simulink model "TST_CoPT_TrqLeadCoord"  (R2016b)
settings: Solver=FixedStepDiscrete  StartTime=0.0  StopTime=simTime  FixedStep=sampleTime  RelTol=1e-3
values from neighbouring files (symbols this model uses):
  testCase = 1    [initTST_CoPT_TrqLeadCoord_001.m]    (also in initTST_CoPT_TrqLeadCoord_002.m = 2)
libraries: simulink x9, UnitTest_Lib x6
settings Model: Creator=zhengjinyan  LastModifiedBy=zhengjinyan
settings DebuggingCC: SignalRangeChecking=error

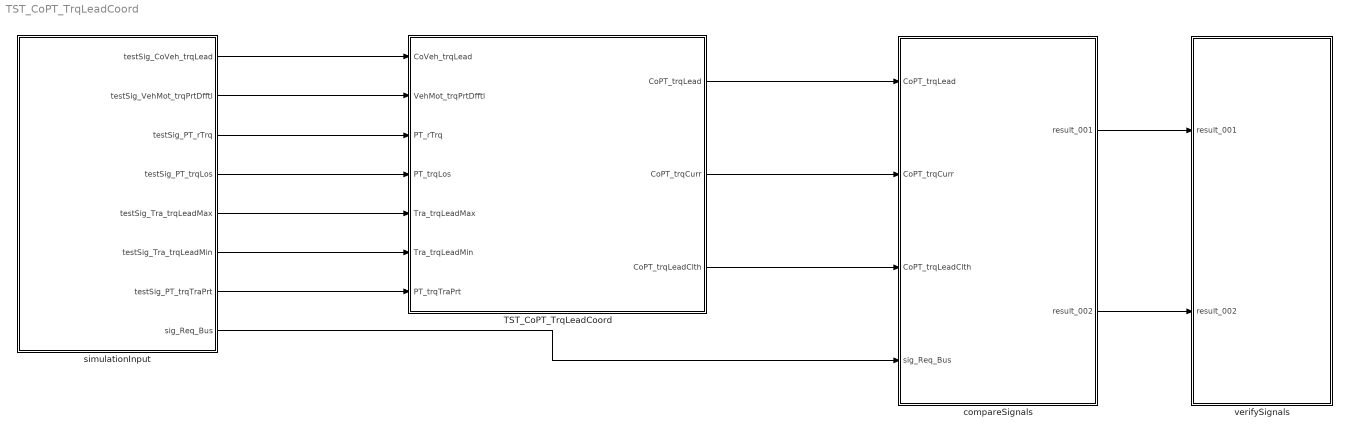
== system TST_CoPT_TrqLeadCoord ==
  TST_CoPT_TrqLeadCoord : Subsystem
  compareSignals : Subsystem
  simulationInput : Subsystem
  verifySignals : Subsystem
  wires:
  simulationInput/1(testSig_CoVeh_trqLead) -> TST_CoPT_TrqLeadCoord/1(CoVeh_trqLead)
  simulationInput/2(testSig_VehMot_trqPrtDfftl) -> TST_CoPT_TrqLeadCoord/2(VehMot_trqPrtDfftl)
  simulationInput/3(testSig_PT_rTrq) -> TST_CoPT_TrqLeadCoord/3(PT_rTrq)
  simulationInput/4(testSig_PT_trqLos) -> TST_CoPT_TrqLeadCoord/4(PT_trqLos)
  simulationInput/5(testSig_Tra_trqLeadMax) -> TST_CoPT_TrqLeadCoord/5(Tra_trqLeadMax)
  simulationInput/6(testSig_Tra_trqLeadMin) -> TST_CoPT_TrqLeadCoord/6(Tra_trqLeadMin)
  simulationInput/7(testSig_PT_trqTraPrt) -> TST_CoPT_TrqLeadCoord/7(PT_trqTraPrt)
  TST_CoPT_TrqLeadCoord/1(CoPT_trqLead) -> compareSignals/1(CoPT_trqLead)
  TST_CoPT_TrqLeadCoord/2(CoPT_trqCurr) -> compareSignals/2(CoPT_trqCurr)
  TST_CoPT_TrqLeadCoord/3(CoPT_trqLeadClth) -> compareSignals/3(CoPT_trqLeadClth)
  simulationInput/8(sig_Req_Bus) -> compareSignals/4(sig_Req_Bus)
  compareSignals/1(result_001) -> verifySignals/1(result_001)
  compareSignals/2(result_002) -> verifySignals/2(result_002)

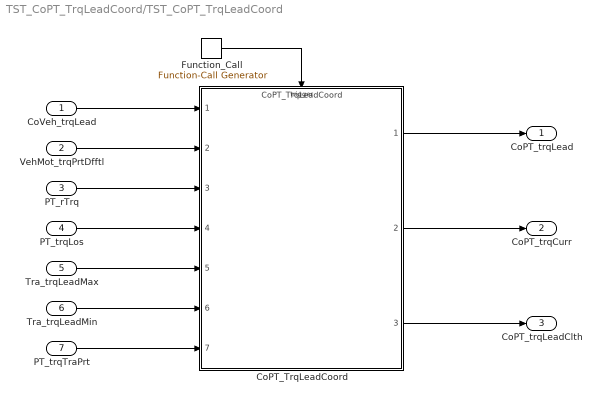
== system TST_CoPT_TrqLeadCoord/TST_CoPT_TrqLeadCoord ==
  CoVeh_trqLead : Inport
  VehMot_trqPrtDfftl : Inport  Port=2
  PT_rTrq : Inport  Port=3
  PT_trqLos : Inport  Port=4
  Tra_trqLeadMax : Inport  Port=5
  Tra_trqLeadMin : Inport  Port=6
  PT_trqTraPrt : Inport  Port=7
  CoPT_TrqLeadCoord : ModelReference  ModelNameDialog=CoPT_TrqLeadCoord  SimulationMode=Normal  ModelReferenceVersion=1.3  TriggerPortName=function  TriggerPortTriggerType=function-call  TriggerPortStatesWhenEnabling=held
  Function_Call : simulink/Ports & Subsystems/Function-Call Generator  sample_time=sampleTime  numberOfIterations=1
  CoPT_trqLead : Outport
  CoPT_trqCurr : Outport  Port=2
  CoPT_trqLeadClth : Outport  Port=3
  wires:
  Function_Call/1 -> CoPT_TrqLeadCoord/Trigger
  CoVeh_trqLead/1 -> CoPT_TrqLeadCoord/1
  VehMot_trqPrtDfftl/1 -> CoPT_TrqLeadCoord/2
  PT_rTrq/1 -> CoPT_TrqLeadCoord/3
  PT_trqLos/1 -> CoPT_TrqLeadCoord/4
  Tra_trqLeadMax/1 -> CoPT_TrqLeadCoord/5
  Tra_trqLeadMin/1 -> CoPT_TrqLeadCoord/6
  PT_trqTraPrt/1 -> CoPT_TrqLeadCoord/7
  CoPT_TrqLeadCoord/1 -> CoPT_trqLead/1
  CoPT_TrqLeadCoord/2 -> CoPT_trqCurr/1
  CoPT_TrqLeadCoord/3 -> CoPT_trqLeadClth/1

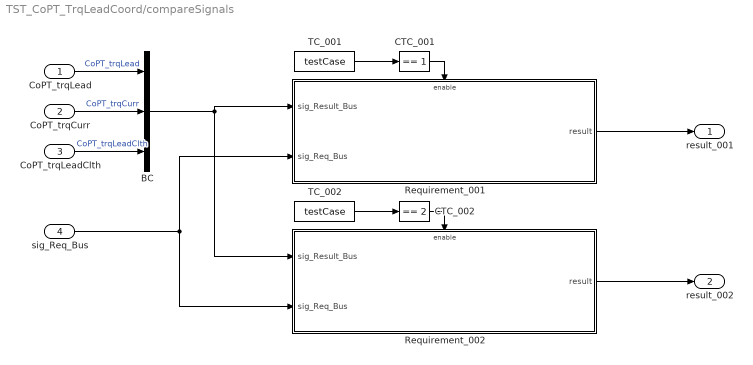
== system TST_CoPT_TrqLeadCoord/compareSignals ==
  CoPT_trqLead : Inport
  CoPT_trqCurr : Inport  Port=2
  CoPT_trqLeadClth : Inport  Port=3
  sig_Req_Bus : Inport  Port=4
  BC : BusCreator  Inputs=3
  CTC_001 : simulink/Logic and Bit Operations/Compare To Constant  relop===  const=1  OutDataTypeStr=boolean
  CTC_002 : simulink/Logic and Bit Operations/Compare To Constant  relop===  const=2  OutDataTypeStr=boolean
  Requirement_001 : Subsystem
  Requirement_002 : Subsystem
  TC_001 : Constant  Value=testCase
  TC_002 : Constant  Value=testCase
  result_001 : Outport
  result_002 : Outport  Port=2
  wires:
  CoPT_trqLead/1 -> BC/1  "CoPT_trqLead"
  CoPT_trqCurr/1 -> BC/2  "CoPT_trqCurr"
  CoPT_trqLeadClth/1 -> BC/3  "CoPT_trqLeadClth"
  TC_001/1 -> CTC_001/1
  CTC_001/1 -> Requirement_001/Enable
  sig_Req_Bus/1 -> Requirement_001/2(sig_Req_Bus), Requirement_002/2(sig_Req_Bus)
  BC/1 -> Requirement_001/1(sig_Result_Bus), Requirement_002/1(sig_Result_Bus)
  Requirement_001/1(result) -> result_001/1
  TC_002/1 -> CTC_002/1
  CTC_002/1 -> Requirement_002/Enable
  Requirement_002/1(result) -> result_002/1

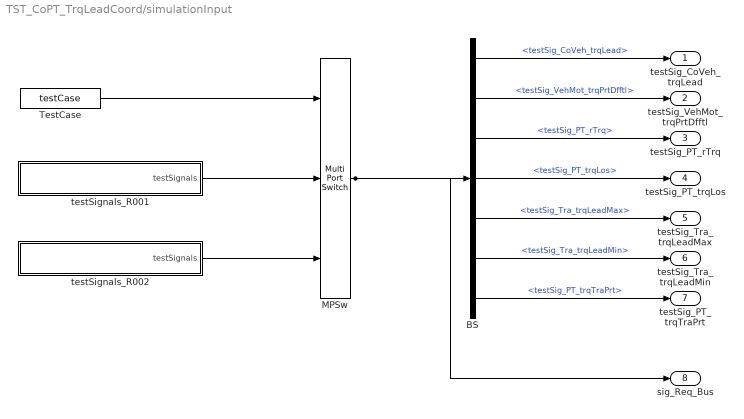
== system TST_CoPT_TrqLeadCoord/simulationInput ==
  BS : BusSelector  OutputSignals=testSig_CoVeh_trqLead,testSig_VehMot_trqPrtDfftl,testSig_PT_rTrq,testSig_PT_trqLos,testSig_Tra_trqLeadMax,testSig_Tra_trqLeadMin,testSig_PT_trqTraPrt
  MPSw : MultiPortSwitch  Inputs=2  SaturateOnIntegerOverflow=on  InputSameDT=on
  TestCase : Constant  Value=testCase
  testSignals_R001 : Subsystem
  testSignals_R002 : Subsystem
  testSig_CoVeh_trqLead : Outport
  testSig_VehMot_trqPrtDfftl : Outport  Port=2
  testSig_PT_rTrq : Outport  Port=3
  testSig_PT_trqLos : Outport  Port=4
  testSig_Tra_trqLeadMax : Outport  Port=5
  testSig_Tra_trqLeadMin : Outport  Port=6
  testSig_PT_trqTraPrt : Outport  Port=7
  sig_Req_Bus : Outport  Port=8
  wires:
  BS/1 -> testSig_CoVeh_trqLead/1  "<testSig_CoVeh_trqLead>"
  BS/2 -> testSig_VehMot_trqPrtDfftl/1  "<testSig_VehMot_trqPrtDfftl>"
  BS/3 -> testSig_PT_rTrq/1  "<testSig_PT_rTrq>"
  BS/4 -> testSig_PT_trqLos/1  "<testSig_PT_trqLos>"
  BS/5 -> testSig_Tra_trqLeadMax/1  "<testSig_Tra_trqLeadMax>"
  BS/6 -> testSig_Tra_trqLeadMin/1  "<testSig_Tra_trqLeadMin>"
  BS/7 -> testSig_PT_trqTraPrt/1  "<testSig_PT_trqTraPrt>"
  MPSw/1 -> BS/1, sig_Req_Bus/1
  TestCase/1 -> MPSw/1
  testSignals_R001/1(testSignals) -> MPSw/2
  testSignals_R002/1(testSignals) -> MPSw/3

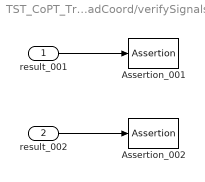
== system TST_CoPT_TrqLeadCoord/verifySignals ==
  result_001 : Inport
  result_002 : Inport  Port=2
  Assertion_001 : Assertion  Enabled=off
  Assertion_002 : Assertion  Enabled=off
  wires:
  result_001/1 -> Assertion_001/1
  result_002/1 -> Assertion_002/1

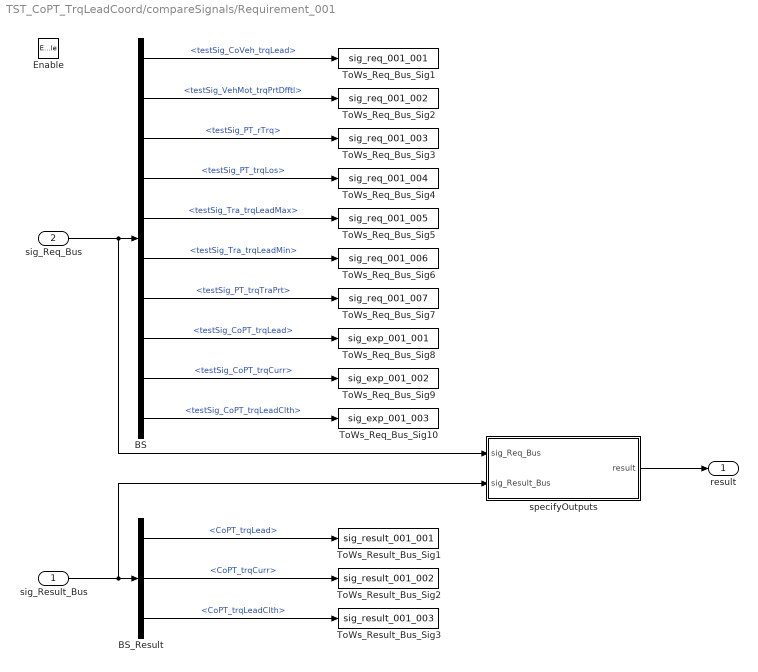
== system TST_CoPT_TrqLeadCoord/compareSignals/Requirement_001 ==
  sig_Result_Bus : Inport
  sig_Req_Bus : Inport  Port=2
  Enable : EnablePort
  BS : BusSelector  OutputSignals=testSig_CoVeh_trqLead,testSig_VehMot_trqPrtDfftl,testSig_PT_rTrq,testSig_PT_trqLos,testSig_Tra_trqLeadMax,testSig_Tra_trqLeadMin,testSig_PT_trqTraPrt,testSig_CoPT_trqLead,testSig_CoPT_trqCurr,testSig_CoPT_trqLeadClth
  BS_Result : BusSelector  OutputSignals=CoPT_trqLead,CoPT_trqCurr,CoPT_trqLeadClth
  ToWs_Req_Bus_Sig1 : ToWorkspace  VariableName=sig_req_001_001  SaveFormat=Structure With Time
  ToWs_Req_Bus_Sig10 : ToWorkspace  VariableName=sig_exp_001_003  SaveFormat=Structure With Time
  ToWs_Req_Bus_Sig2 : ToWorkspace  VariableName=sig_req_001_002  SaveFormat=Structure With Time
  ToWs_Req_Bus_Sig3 : ToWorkspace  VariableName=sig_req_001_003  SaveFormat=Structure With Time
  ToWs_Req_Bus_Sig4 : ToWorkspace  VariableName=sig_req_001_004  SaveFormat=Structure With Time
  ToWs_Req_Bus_Sig5 : ToWorkspace  VariableName=sig_req_001_005  SaveFormat=Structure With Time
  ToWs_Req_Bus_Sig6 : ToWorkspace  VariableName=sig_req_001_006  SaveFormat=Structure With Time
  ToWs_Req_Bus_Sig7 : ToWorkspace  VariableName=sig_req_001_007  SaveFormat=Structure With Time
  ToWs_Req_Bus_Sig8 : ToWorkspace  VariableName=sig_exp_001_001  SaveFormat=Structure With Time
  ToWs_Req_Bus_Sig9 : ToWorkspace  VariableName=sig_exp_001_002  SaveFormat=Structure With Time
  ToWs_Result_Bus_Sig1 : ToWorkspace  VariableName=sig_result_001_001  SaveFormat=Structure With Time
  ToWs_Result_Bus_Sig2 : ToWorkspace  VariableName=sig_result_001_002  SaveFormat=Structure With Time
  ToWs_Result_Bus_Sig3 : ToWorkspace  VariableName=sig_result_001_003  SaveFormat=Structure With Time
  specifyOutputs : Subsystem
  result : Outport
  wires:
  sig_Req_Bus/1 -> BS/1, specifyOutputs/1(sig_Req_Bus)
  BS/1 -> ToWs_Req_Bus_Sig1/1  "<testSig_CoVeh_trqLead>"
  BS/2 -> ToWs_Req_Bus_Sig2/1  "<testSig_VehMot_trqPrtDfftl>"
  BS/3 -> ToWs_Req_Bus_Sig3/1  "<testSig_PT_rTrq>"
  BS/4 -> ToWs_Req_Bus_Sig4/1  "<testSig_PT_trqLos>"
  BS/5 -> ToWs_Req_Bus_Sig5/1  "<testSig_Tra_trqLeadMax>"
  BS/6 -> ToWs_Req_Bus_Sig6/1  "<testSig_Tra_trqLeadMin>"
  BS/7 -> ToWs_Req_Bus_Sig7/1  "<testSig_PT_trqTraPrt>"
  BS/8 -> ToWs_Req_Bus_Sig8/1  "<testSig_CoPT_trqLead>"
  BS/9 -> ToWs_Req_Bus_Sig9/1  "<testSig_CoPT_trqCurr>"
  BS/10 -> ToWs_Req_Bus_Sig10/1  "<testSig_CoPT_trqLeadClth>"
  sig_Result_Bus/1 -> BS_Result/1, specifyOutputs/2(sig_Result_Bus)
  BS_Result/1 -> ToWs_Result_Bus_Sig1/1  "<CoPT_trqLead>"
  BS_Result/2 -> ToWs_Result_Bus_Sig2/1  "<CoPT_trqCurr>"
  BS_Result/3 -> ToWs_Result_Bus_Sig3/1  "<CoPT_trqLeadClth>"
  specifyOutputs/1(result) -> result/1

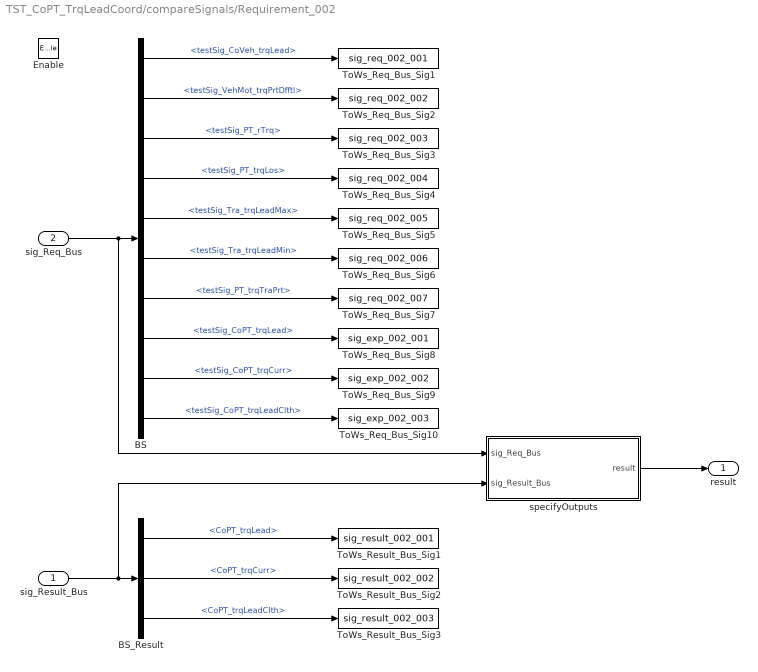
== system TST_CoPT_TrqLeadCoord/compareSignals/Requirement_002 ==
  sig_Result_Bus : Inport
  sig_Req_Bus : Inport  Port=2
  Enable : EnablePort
  BS : BusSelector  OutputSignals=testSig_CoVeh_trqLead,testSig_VehMot_trqPrtDfftl,testSig_PT_rTrq,testSig_PT_trqLos,testSig_Tra_trqLeadMax,testSig_Tra_trqLeadMin,testSig_PT_trqTraPrt,testSig_CoPT_trqLead,testSig_CoPT_trqCurr,testSig_CoPT_trqLeadClth
  BS_Result : BusSelector  OutputSignals=CoPT_trqLead,CoPT_trqCurr,CoPT_trqLeadClth
  ToWs_Req_Bus_Sig1 : ToWorkspace  VariableName=sig_req_002_001  SaveFormat=Structure With Time
  ToWs_Req_Bus_Sig10 : ToWorkspace  VariableName=sig_exp_002_003  SaveFormat=Structure With Time
  ToWs_Req_Bus_Sig2 : ToWorkspace  VariableName=sig_req_002_002  SaveFormat=Structure With Time
  ToWs_Req_Bus_Sig3 : ToWorkspace  VariableName=sig_req_002_003  SaveFormat=Structure With Time
  ToWs_Req_Bus_Sig4 : ToWorkspace  VariableName=sig_req_002_004  SaveFormat=Structure With Time
  ToWs_Req_Bus_Sig5 : ToWorkspace  VariableName=sig_req_002_005  SaveFormat=Structure With Time
  ToWs_Req_Bus_Sig6 : ToWorkspace  VariableName=sig_req_002_006  SaveFormat=Structure With Time
  ToWs_Req_Bus_Sig7 : ToWorkspace  VariableName=sig_req_002_007  SaveFormat=Structure With Time
  ToWs_Req_Bus_Sig8 : ToWorkspace  VariableName=sig_exp_002_001  SaveFormat=Structure With Time
  ToWs_Req_Bus_Sig9 : ToWorkspace  VariableName=sig_exp_002_002  SaveFormat=Structure With Time
  ToWs_Result_Bus_Sig1 : ToWorkspace  VariableName=sig_result_002_001  SaveFormat=Structure With Time
  ToWs_Result_Bus_Sig2 : ToWorkspace  VariableName=sig_result_002_002  SaveFormat=Structure With Time
  ToWs_Result_Bus_Sig3 : ToWorkspace  VariableName=sig_result_002_003  SaveFormat=Structure With Time
  specifyOutputs : Subsystem
  result : Outport
  wires:
  sig_Req_Bus/1 -> BS/1, specifyOutputs/1(sig_Req_Bus)
  BS/1 -> ToWs_Req_Bus_Sig1/1  "<testSig_CoVeh_trqLead>"
  BS/2 -> ToWs_Req_Bus_Sig2/1  "<testSig_VehMot_trqPrtDfftl>"
  BS/3 -> ToWs_Req_Bus_Sig3/1  "<testSig_PT_rTrq>"
  BS/4 -> ToWs_Req_Bus_Sig4/1  "<testSig_PT_trqLos>"
  BS/5 -> ToWs_Req_Bus_Sig5/1  "<testSig_Tra_trqLeadMax>"
  BS/6 -> ToWs_Req_Bus_Sig6/1  "<testSig_Tra_trqLeadMin>"
  BS/7 -> ToWs_Req_Bus_Sig7/1  "<testSig_PT_trqTraPrt>"
  BS/8 -> ToWs_Req_Bus_Sig8/1  "<testSig_CoPT_trqLead>"
  BS/9 -> ToWs_Req_Bus_Sig9/1  "<testSig_CoPT_trqCurr>"
  BS/10 -> ToWs_Req_Bus_Sig10/1  "<testSig_CoPT_trqLeadClth>"
  sig_Result_Bus/1 -> BS_Result/1, specifyOutputs/2(sig_Result_Bus)
  BS_Result/1 -> ToWs_Result_Bus_Sig1/1  "<CoPT_trqLead>"
  BS_Result/2 -> ToWs_Result_Bus_Sig2/1  "<CoPT_trqCurr>"
  BS_Result/3 -> ToWs_Result_Bus_Sig3/1  "<CoPT_trqLeadClth>"
  specifyOutputs/1(result) -> result/1

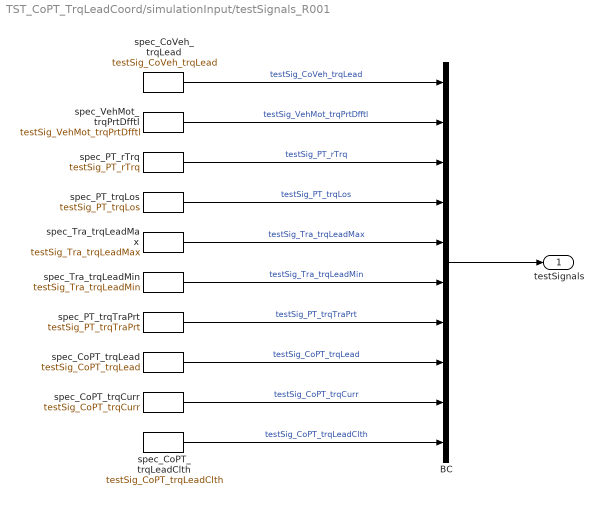
== system TST_CoPT_TrqLeadCoord/simulationInput/testSignals_R001 ==
  BC : BusCreator  Inputs=10
  spec_CoPT_trqCurr : FromWorkspace  VariableName=testSig_CoPT_trqCurr  Interpolate=off  OutputAfterFinalValue=Holding final value
  spec_CoPT_trqLead : FromWorkspace  VariableName=testSig_CoPT_trqLead  Interpolate=off  OutputAfterFinalValue=Holding final value
  spec_CoPT_trqLeadClth : FromWorkspace  VariableName=testSig_CoPT_trqLeadClth  Interpolate=off  OutputAfterFinalValue=Holding final value
  spec_CoVeh_trqLead : FromWorkspace  VariableName=testSig_CoVeh_trqLead  Interpolate=off  OutputAfterFinalValue=Holding final value
  spec_PT_rTrq : FromWorkspace  VariableName=testSig_PT_rTrq  Interpolate=off  OutputAfterFinalValue=Holding final value
  spec_PT_trqLos : FromWorkspace  VariableName=testSig_PT_trqLos  Interpolate=off  OutputAfterFinalValue=Holding final value
  spec_PT_trqTraPrt : FromWorkspace  VariableName=testSig_PT_trqTraPrt  Interpolate=off  OutputAfterFinalValue=Holding final value
  spec_Tra_trqLeadMax : FromWorkspace  VariableName=testSig_Tra_trqLeadMax  Interpolate=off  OutputAfterFinalValue=Holding final value
  spec_Tra_trqLeadMin : FromWorkspace  VariableName=testSig_Tra_trqLeadMin  Interpolate=off  OutputAfterFinalValue=Holding final value
  spec_VehMot_trqPrtDfftl : FromWorkspace  VariableName=testSig_VehMot_trqPrtDfftl  Interpolate=off  OutputAfterFinalValue=Holding final value
  testSignals : Outport
  wires:
  BC/1 -> testSignals/1
  spec_CoVeh_trqLead/1 -> BC/1  "testSig_CoVeh_trqLead"
  spec_VehMot_trqPrtDfftl/1 -> BC/2  "testSig_VehMot_trqPrtDfftl"
  spec_PT_rTrq/1 -> BC/3  "testSig_PT_rTrq"
  spec_PT_trqLos/1 -> BC/4  "testSig_PT_trqLos"
  spec_Tra_trqLeadMax/1 -> BC/5  "testSig_Tra_trqLeadMax"
  spec_Tra_trqLeadMin/1 -> BC/6  "testSig_Tra_trqLeadMin"
  spec_PT_trqTraPrt/1 -> BC/7  "testSig_PT_trqTraPrt"
  spec_CoPT_trqLead/1 -> BC/8  "testSig_CoPT_trqLead"
  spec_CoPT_trqCurr/1 -> BC/9  "testSig_CoPT_trqCurr"
  spec_CoPT_trqLeadClth/1 -> BC/10  "testSig_CoPT_trqLeadClth"

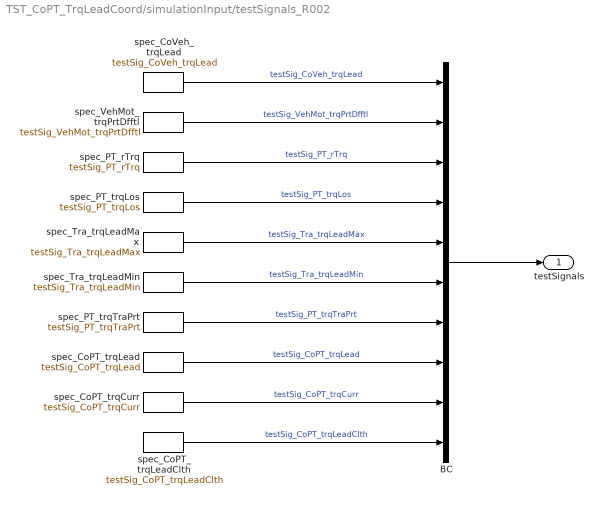
== system TST_CoPT_TrqLeadCoord/simulationInput/testSignals_R002 ==
  BC : BusCreator  Inputs=10
  spec_CoPT_trqCurr : FromWorkspace  VariableName=testSig_CoPT_trqCurr  Interpolate=off  OutputAfterFinalValue=Holding final value
  spec_CoPT_trqLead : FromWorkspace  VariableName=testSig_CoPT_trqLead  Interpolate=off  OutputAfterFinalValue=Holding final value
  spec_CoPT_trqLeadClth : FromWorkspace  VariableName=testSig_CoPT_trqLeadClth  Interpolate=off  OutputAfterFinalValue=Holding final value
  spec_CoVeh_trqLead : FromWorkspace  VariableName=testSig_CoVeh_trqLead  Interpolate=off  OutputAfterFinalValue=Holding final value
  spec_PT_rTrq : FromWorkspace  VariableName=testSig_PT_rTrq  Interpolate=off  OutputAfterFinalValue=Holding final value
  spec_PT_trqLos : FromWorkspace  VariableName=testSig_PT_trqLos  Interpolate=off  OutputAfterFinalValue=Holding final value
  spec_PT_trqTraPrt : FromWorkspace  VariableName=testSig_PT_trqTraPrt  Interpolate=off  OutputAfterFinalValue=Holding final value
  spec_Tra_trqLeadMax : FromWorkspace  VariableName=testSig_Tra_trqLeadMax  Interpolate=off  OutputAfterFinalValue=Holding final value
  spec_Tra_trqLeadMin : FromWorkspace  VariableName=testSig_Tra_trqLeadMin  Interpolate=off  OutputAfterFinalValue=Holding final value
  spec_VehMot_trqPrtDfftl : FromWorkspace  VariableName=testSig_VehMot_trqPrtDfftl  Interpolate=off  OutputAfterFinalValue=Holding final value
  testSignals : Outport
  wires:
  BC/1 -> testSignals/1
  spec_CoVeh_trqLead/1 -> BC/1  "testSig_CoVeh_trqLead"
  spec_VehMot_trqPrtDfftl/1 -> BC/2  "testSig_VehMot_trqPrtDfftl"
  spec_PT_rTrq/1 -> BC/3  "testSig_PT_rTrq"
  spec_PT_trqLos/1 -> BC/4  "testSig_PT_trqLos"
  spec_Tra_trqLeadMax/1 -> BC/5  "testSig_Tra_trqLeadMax"
  spec_Tra_trqLeadMin/1 -> BC/6  "testSig_Tra_trqLeadMin"
  spec_PT_trqTraPrt/1 -> BC/7  "testSig_PT_trqTraPrt"
  spec_CoPT_trqLead/1 -> BC/8  "testSig_CoPT_trqLead"
  spec_CoPT_trqCurr/1 -> BC/9  "testSig_CoPT_trqCurr"
  spec_CoPT_trqLeadClth/1 -> BC/10  "testSig_CoPT_trqLeadClth"

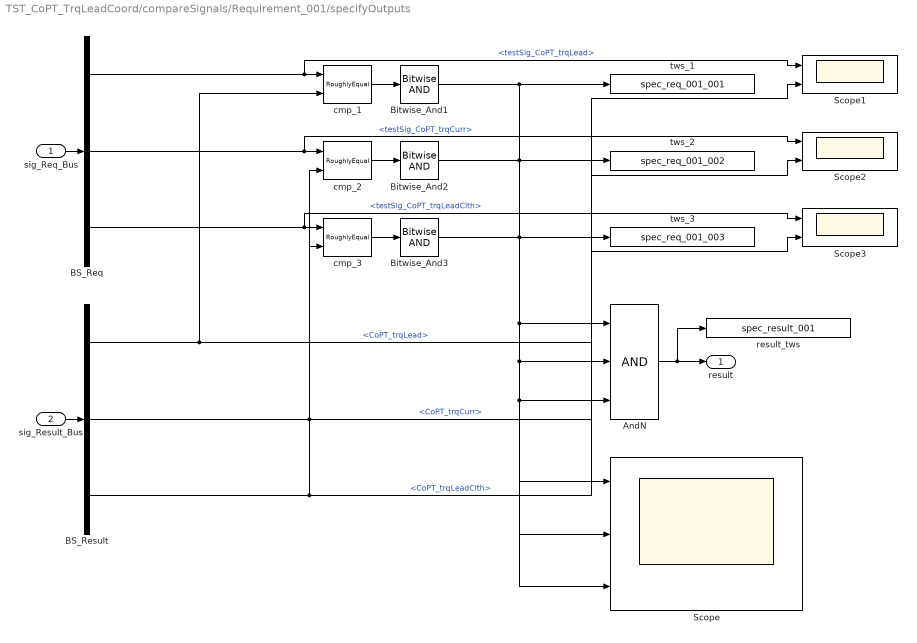
== system TST_CoPT_TrqLeadCoord/compareSignals/Requirement_001/specifyOutputs ==
  sig_Req_Bus : Inport
  sig_Result_Bus : Inport  Port=2
  AndN : Logic  Inputs=3
  BS_Req : BusSelector  OutputSignals=testSig_CoPT_trqLead,testSig_CoPT_trqCurr,testSig_CoPT_trqLeadClth
  BS_Result : BusSelector  OutputSignals=CoPT_trqLead,CoPT_trqCurr,CoPT_trqLeadClth
  Bitwise_And1 : simulink/Logic and Bit Operations/Bitwise Operator  logicop=AND  UseBitMask=off  BitMask=bin2dec('11011001')  BitMaskRealWorld=Stored Integer
  Bitwise_And2 : simulink/Logic and Bit Operations/Bitwise Operator  logicop=AND  UseBitMask=off  BitMask=bin2dec('11011001')  BitMaskRealWorld=Stored Integer
  Bitwise_And3 : simulink/Logic and Bit Operations/Bitwise Operator  logicop=AND  UseBitMask=off  BitMask=bin2dec('11011001')  BitMaskRealWorld=Stored Integer
  Scope : Scope  NumInputPorts=3
  Scope1 : Scope  NumInputPorts=2
  Scope2 : Scope  NumInputPorts=2
  Scope3 : Scope  NumInputPorts=2
  cmp_1 : UnitTest_Lib/RoughlyEqual  slope=0.5
  cmp_2 : UnitTest_Lib/RoughlyEqual  slope=0.5
  cmp_3 : UnitTest_Lib/RoughlyEqual  slope=0.1
  result_tws : ToWorkspace  VariableName=spec_result_001
  tws_1 : ToWorkspace  VariableName=spec_req_001_001
  tws_2 : ToWorkspace  VariableName=spec_req_001_002
  tws_3 : ToWorkspace  VariableName=spec_req_001_003
  result : Outport
  wires:
  sig_Req_Bus/1 -> BS_Req/1
  sig_Result_Bus/1 -> BS_Result/1
  AndN/1 -> result/1, result_tws/1
  BS_Req/1 -> cmp_1/1, Scope1/1  "<testSig_CoPT_trqLead>"
  BS_Result/1 -> cmp_1/2, Scope1/2  "<CoPT_trqLead>"
  cmp_1/1 -> Bitwise_And1/1
  Bitwise_And1/1 -> AndN/1, Scope/1, tws_1/1
  BS_Req/2 -> cmp_2/1, Scope2/1  "<testSig_CoPT_trqCurr>"
  BS_Result/2 -> cmp_2/2, Scope2/2  "<CoPT_trqCurr>"
  cmp_2/1 -> Bitwise_And2/1
  Bitwise_And2/1 -> AndN/2, Scope/2, tws_2/1
  BS_Req/3 -> cmp_3/1, Scope3/1  "<testSig_CoPT_trqLeadClth>"
  BS_Result/3 -> cmp_3/2, Scope3/2  "<CoPT_trqLeadClth>"
  cmp_3/1 -> Bitwise_And3/1
  Bitwise_And3/1 -> AndN/3, Scope/3, tws_3/1

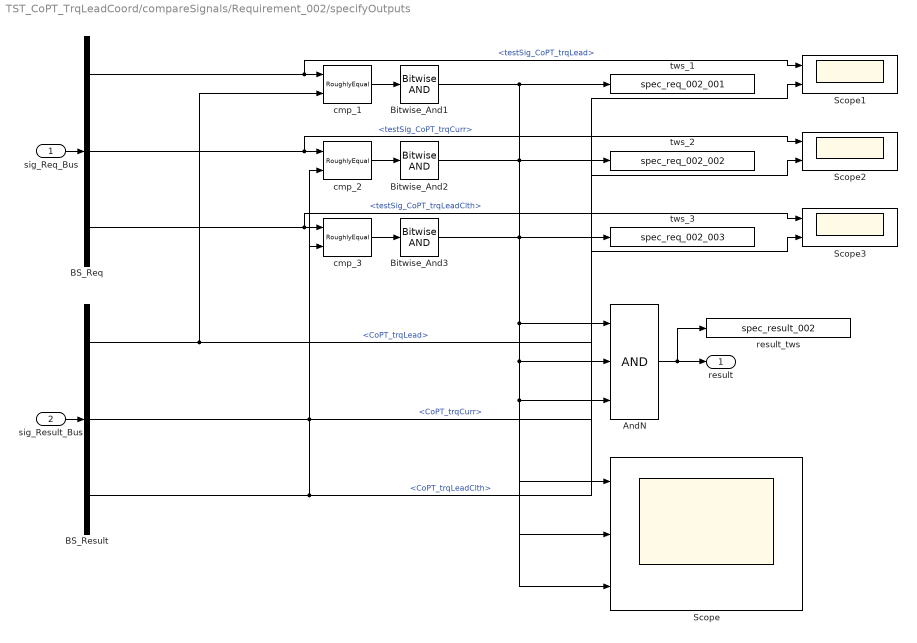
== system TST_CoPT_TrqLeadCoord/compareSignals/Requirement_002/specifyOutputs ==
  sig_Req_Bus : Inport
  sig_Result_Bus : Inport  Port=2
  AndN : Logic  Inputs=3
  BS_Req : BusSelector  OutputSignals=testSig_CoPT_trqLead,testSig_CoPT_trqCurr,testSig_CoPT_trqLeadClth
  BS_Result : BusSelector  OutputSignals=CoPT_trqLead,CoPT_trqCurr,CoPT_trqLeadClth
  Bitwise_And1 : simulink/Logic and Bit Operations/Bitwise Operator  logicop=AND  UseBitMask=off  BitMask=bin2dec('11011001')  BitMaskRealWorld=Stored Integer
  Bitwise_And2 : simulink/Logic and Bit Operations/Bitwise Operator  logicop=AND  UseBitMask=off  BitMask=bin2dec('11011001')  BitMaskRealWorld=Stored Integer
  Bitwise_And3 : simulink/Logic and Bit Operations/Bitwise Operator  logicop=AND  UseBitMask=off  BitMask=bin2dec('11011001')  BitMaskRealWorld=Stored Integer
  Scope : Scope  NumInputPorts=3
  Scope1 : Scope  NumInputPorts=2
  Scope2 : Scope  NumInputPorts=2
  Scope3 : Scope  NumInputPorts=2
  cmp_1 : UnitTest_Lib/RoughlyEqual  slope=0.5
  cmp_2 : UnitTest_Lib/RoughlyEqual  slope=0.5
  cmp_3 : UnitTest_Lib/RoughlyEqual  slope=0.1
  result_tws : ToWorkspace  VariableName=spec_result_002
  tws_1 : ToWorkspace  VariableName=spec_req_002_001
  tws_2 : ToWorkspace  VariableName=spec_req_002_002
  tws_3 : ToWorkspace  VariableName=spec_req_002_003
  result : Outport
  wires:
  sig_Req_Bus/1 -> BS_Req/1
  sig_Result_Bus/1 -> BS_Result/1
  AndN/1 -> result/1, result_tws/1
  BS_Req/1 -> cmp_1/1, Scope1/1  "<testSig_CoPT_trqLead>"
  BS_Result/1 -> cmp_1/2, Scope1/2  "<CoPT_trqLead>"
  cmp_1/1 -> Bitwise_And1/1
  Bitwise_And1/1 -> AndN/1, Scope/1, tws_1/1
  BS_Req/2 -> cmp_2/1, Scope2/1  "<testSig_CoPT_trqCurr>"
  BS_Result/2 -> cmp_2/2, Scope2/2  "<CoPT_trqCurr>"
  cmp_2/1 -> Bitwise_And2/1
  Bitwise_And2/1 -> AndN/2, Scope/2, tws_2/1
  BS_Req/3 -> cmp_3/1, Scope3/1  "<testSig_CoPT_trqLeadClth>"
  BS_Result/3 -> cmp_3/2, Scope3/2  "<CoPT_trqLeadClth>"
  cmp_3/1 -> Bitwise_And3/1
  Bitwise_And3/1 -> AndN/3, Scope/3, tws_3/1
